simulink model "blockdemo"  (Simulink 6.3)
settings: Solver=VariableStepDiscrete  StartTime=0.0  StopTime=1E-6  RelTol=1e-3
InitFcn:
  | %% DSPBuilder Start
  | alt_dspbuilder_update_model(bdroot)
  | %% DSPBuilder End
libraries: allblocks_alteradspbuilder2 x15, simulink x2
settings Model: Creator=cpurcell  LastModifiedBy=delphick
settings DebuggingCC: MultiTaskDSMMsg=error

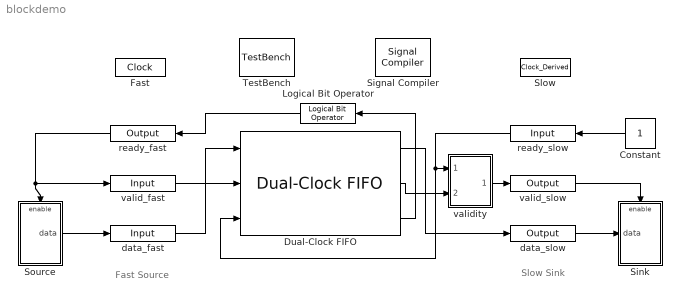
== system blockdemo ==
  note: Fast Source
  note: Slow Sink
  Constant : Constant  Orientation=left
  Dual-Clock FIFO : allblocks_alteradspbuilder2/Dual-Clock FIFO  numwords=64  BusType=Signed Integer  bwl=8  bwr=0  ram_type=AUTO  UseBaseWriteClock=off  write_clock=Fast  UseBaseReadClock=off  read_clock=Slow  use_rdempty=on  use_rdfull=off  use_rdusedw=off  use_wrempty=off  use_wrfull=on  use_wrusedw=off  use_user_aclr=off  register_output=off  use_les_only=off  showahead_mode=off  synchronized=off
  Fast : allblocks_alteradspbuilder2/Clock  ClockPeriod=20  ClockPeriodUnit=ns  SampleTime=20e-9  SimulationStartCycle=5  PhaseOffset=0  Reset=aclr_fast  Export=off
  Logical Bit Operator : allblocks_alteradspbuilder2/Logical Bit Operator  Orientation=left  LogicalOperator=NOT  user_inputs=2
  Signal Compiler : allblocks_alteradspbuilder2/Signal Compiler  DeviceFamily=Stratix III  DeviceName=AUTO  EnableSignalTap=off  SignalTapDepth=128  UseBoardBlock=off  StpUseDefaultClock=on  StpClock=Fast
  Sink : Subsystem
  Slow : allblocks_alteradspbuilder2/Clock_Derived  ClockNumerator=2  ClockDenominator=1  SimulationStartCycle=5  PhaseOffset=0  Reset=aclr_slow  Export=off
  Source : Subsystem
  TestBench : allblocks_alteradspbuilder2/TestBench  enable=on  advancedMode=off  modelSimGui=off  simdatafile=C:\workspace_clean\Documentation\DesignExamples\Tutorials\UnitBlocks\Storage\DualClockFIFO\tb_blockdemo\blockdemo.simdata.tcl
  data_fast : allblocks_alteradspbuilder2/Input  iofile=C:\workspace_clean\Documentation\DesignExamples\Tutorials\UnitBlocks\Storage\DualClockFIFO\tb_blockdemo\blockdemo_data_fast.salt  BusType=Signed Integer  bwl=8  bwr=0  SpecifyClock=on  clock=Fast  PORTTYPE=Input
  data_slow : allblocks_alteradspbuilder2/Output  iofile=C:\workspace_clean\Documentation\DesignExamples\Tutorials\UnitBlocks\Storage\DualClockFIFO\tb_blockdemo\blockdemo_data_slow.capture  BusType=Signed Integer  bwl=8  bwr=0  PORTTYPE=Output
  ready_fast : allblocks_alteradspbuilder2/Output  Orientation=left  iofile=C:\workspace_clean\Documentation\DesignExamples\Tutorials\UnitBlocks\Storage\DualClockFIFO\tb_blockdemo\blockdemo_ready_fast.capture  BusType=Single Bit  bwl=8  bwr=0  PORTTYPE=Output
  ready_slow : allblocks_alteradspbuilder2/Input  Orientation=left  iofile=C:\workspace_clean\Documentation\DesignExamples\Tutorials\UnitBlocks\Storage\DualClockFIFO\tb_blockdemo\blockdemo_ready_slow.salt  BusType=Single Bit  bwl=8  bwr=0  SpecifyClock=on  clock=Slow  PORTTYPE=Input
  valid_fast : allblocks_alteradspbuilder2/Input  iofile=C:\workspace_clean\Documentation\DesignExamples\Tutorials\UnitBlocks\Storage\DualClockFIFO\tb_blockdemo\blockdemo_valid_fast.salt  BusType=Single Bit  bwl=8  bwr=0  SpecifyClock=on  clock=Fast  PORTTYPE=Input
  valid_slow : allblocks_alteradspbuilder2/Output  iofile=C:\workspace_clean\Documentation\DesignExamples\Tutorials\UnitBlocks\Storage\DualClockFIFO\tb_blockdemo\blockdemo_valid_slow.capture  BusType=Single Bit  bwl=8  bwr=0  PORTTYPE=Output
  validity : Subsystem
  wires:
  data_fast/1 -> Dual-Clock FIFO/1
  valid_fast/1 -> Dual-Clock FIFO/2
  Dual-Clock FIFO/3 -> Logical Bit Operator/1
  Logical Bit Operator/1 -> ready_fast/1
  ready_slow/1 -> Dual-Clock FIFO/3, validity/1(empty)
  Dual-Clock FIFO/1 -> data_slow/1
  Source/1(data) -> data_fast/1
  ready_fast/1 -> Source/Enable, valid_fast/1
  Constant/1 -> ready_slow/1
  validity/1(valid) -> valid_slow/1
  data_slow/1 -> Sink/1(data)
  valid_slow/1 -> Sink/Enable
  Dual-Clock FIFO/2 -> validity/2(ready)

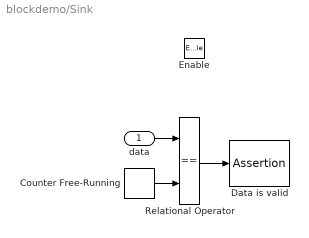
== system blockdemo/Sink ==
  data : Inport
  Enable : EnablePort
  Counter Free-Running : simulink/Sources/Counter Free-Running  SystemSampleTime=-1  NumBits=32  tsamp=-1
  Data is valid : Assertion
  Relational Operator : RelationalOperator  Operator===  LogicOutDataTypeMode=Boolean
  wires:
  Counter Free-Running/1 -> Relational Operator/2
  data/1 -> Relational Operator/1
  Relational Operator/1 -> Data is valid/1

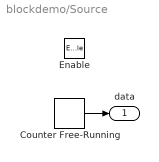
== system blockdemo/Source ==
  Enable : EnablePort
  Counter Free-Running : simulink/Sources/Counter Free-Running  SystemSampleTime=-1  NumBits=32  tsamp=-1
  data : Outport  InitialOutput=0
  wires:
  Counter Free-Running/1 -> data/1

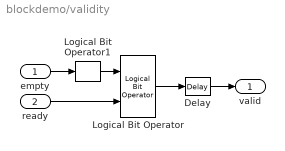
== system blockdemo/validity ==
  empty : Inport
  ready : Inport  Port=2
  Delay : allblocks_alteradspbuilder2/Delay  pipeline=1  ClockPhase=1  use_ena=off  use_sclr=off
  Logical Bit Operator : allblocks_alteradspbuilder2/Logical Bit Operator  LogicalOperator=AND  user_inputs=2
  Logical Bit Operator1 : allblocks_alteradspbuilder2/Logical Bit Operator  LogicalOperator=NOT  user_inputs=2
  valid : Outport
  wires:
  Delay/1 -> valid/1
  empty/1 -> Logical Bit Operator1/1
  Logical Bit Operator/1 -> Delay/1
  Logical Bit Operator1/1 -> Logical Bit Operator/1
  ready/1 -> Logical Bit Operator/2
